simulink model "simulation_LQI"  (R2021b)
settings: Solver=FixedStepAuto  StartTime=0.0  StopTime=T  RelTol=1e-3  EnableMultiTasking=on
undefined symbols (not defined in the file or in its folder): DiscIntNeverNeededParam, discrete_eq, h, Humusoft, K_qli, MF634
libraries: sldrtlib x2, eeLuenbergerObserver x1, simulink x1
settings Model: Creator=rbabuska  LastModifiedBy=wterhaar
settings SolverCC: AlgebraicLoopSolver=TrustRegion  AutoInsertRateTranBlk=on
settings DataIOCC: LimitDataPoints=on  SaveFormat=Array  SignalLoggingSaveFormat=ModelDataLogs  SaveOutput=off  SaveTime=off  ReturnWorkspaceOutputs=off
settings OptimizationCC: DefaultParameterBehavior=Inlined  InlineInvariantSignals=on  EnhancedBackFolding=on  PassReuseOutputArgsAs=Individual arguments  ExpressionDepthLimit=2147483647  StateBitsets=on  DataBitsets=on  ZeroExternalMemoryAtStartup=off  ZeroInternalMemoryAtStartup=off  NoFixptDivByZeroProtection=on  LifeSpan=1  OptimizeBlockOrder=speed  DifferentSizesBufferReuse=on  EfficientTunableParamExpr=on
settings DebuggingCC: UnderspecifiedInitializationDetection=Classic  MergeDetectMultiDrivingBlocksExec=none  ParameterTunabilityLossMsg=error  FcnCallInpInsideContextMsg=warning  StateNameClashWarn=warning  SFUnexpectedBacktrackingDiag=warning  SFNoUnconditionalDefaultTransitionDiag=warning  SFExecutionAtInitializationDiag=none  SFMachineParentedDataDiag=warning  ArithmeticOperatorsInVariantConditions=warning
settings HardwareCC: ProdBitPerPointer=32  ProdBitPerSizeT=32  ProdBitPerPtrDiffT=32  ProdLargestAtomicFloat=None  ProdIntDivRoundTo=Floor  ProdWordSize=32  ProdHWDeviceType=Generic->Custom
settings ModelReferenceCC: PropagateSignalLabelsOutOfModel=off
settings SFSimCC: SimUseLocalCustomCode=off  MATLABDynamicMemAlloc=off  CustomCodeUndefinedFunction=UseInterfaceOnly
settings RTWCC: Description=Embedded Coder  SystemTargetFile=ert.tlc  TLCOptions=-p0  GenCodeOnly=on  TemplateMakefile=ert_default_tmf  GenerateReport=on  RTWVerbose=off  RTWUseLocalCustomCode=off  IncludeHyperlinkInReport=on  LaunchReport=on
settings CodeAppCC: ForceParamTrailComments=on  IgnoreCustomStorageClasses=off  OperatorAnnotations=on  SimulinkDataObjDesc=on  SFDataObjDesc=on  CustomSymbolStrGlobalVar=rt$N$M  CustomSymbolStrType=$N$M  CustomSymbolStrFcn=$N$M$F  CustomSymbolStrMacro=$N$M  InsertBlockDesc=on
settings ERTTargetCC: CodeReplacementLibrary=ISO_C  GenerateSampleERTMain=on  IncludeMdlTerminateFcn=off  SuppressErrorStatus=on  SupportAbsoluteTime=off  PurelyIntegerCode=on  SupportNonFinite=off  SupportComplex=off  InlinedParameterPlacement=NonHierarchical  RootIOFormat=Structure reference  ERTCustomFileTemplate=example_file_process.tlc
settings ConfigComp: CovMetricSettings=dw  CovSaveCumulativeToWorkspaceVar=on  CovSaveSingleToWorkspaceVar=on  CovExternalEMLEnable=off  CovSFcnEnable=off

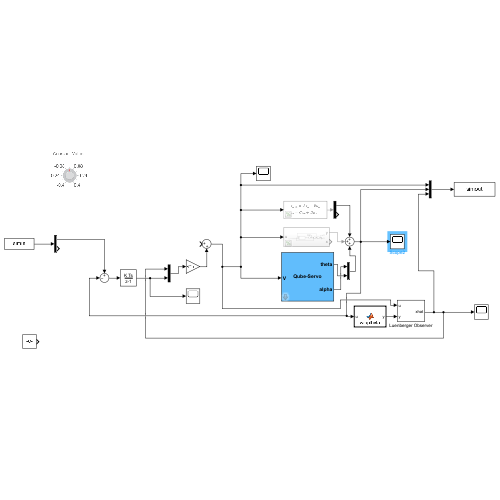
[thumbnail: Simulink's stored preview of the top-level diagram]
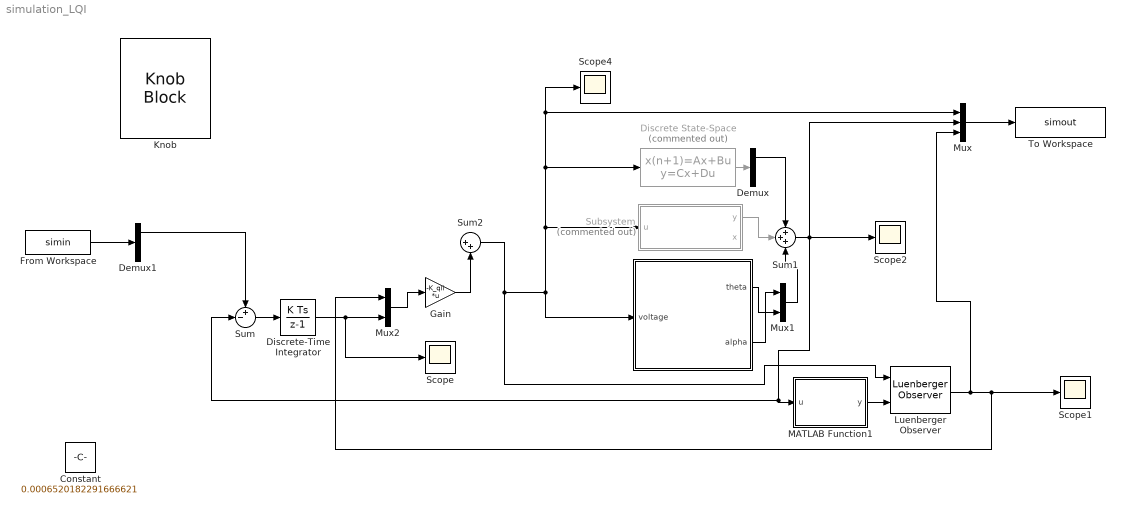
== system simulation_LQI ==
  " " : Subsystem  LoadFcn=hwinit  InitFcn=hwinit  mask{h=h}
      mask prompts: h "Sampling period [s]"
      mask Display:
      | disp('Qube-Servo')
      | port_label('output',1,'theta')
      | port_label('output',2,'alpha')
      | port_label('input',1,'V')
  Constant : Constant  Value=0.0006520182291666621
  Demux : Demux  Outputs=[2;4]
  Demux1 : Demux  Outputs=[2 2]
  Discrete State-Space : DiscreteStateSpace  Commented=on  A=discrete_eq.A  B=discrete_eq.B  C=[discrete_eq.C;eye(4)]  D=[discrete_eq.D;zeros(4,1)]  InitialCondition=[0;0;0;0]  SampleTime=h
  Discrete-Time Integrator : DiscreteIntegrator  gainval=[1;0.001]  InitialCondition=[0;0]  SampleTime=h  ICPrevOutput=DiscIntNeverNeededParam  ICPrevScaledInput=DiscIntNeverNeededParam
  From Workspace : FromWorkspace  VariableName=simin  SampleTime=h  OutputAfterFinalValue=Holding final value
  Gain : Gain  Gain=-K_qli  Multiplication=Matrix(K*u)
  Knob : KnobBlock  ScaleMin=-0.4  ScaleMax=0.4
  Luenberger Observer : eeLuenbergerObserver/Luenberger Observer  StateSpaceType=Discrete-time  Ad=discrete_eq.A  Bd=discrete_eq.B  Cd=discrete_eq.C  Dd=discrete_eq.D  A=1  B=1  C=1  D=1  ObserverDesign=Observer gain  Ld=disc  DesiredEigenvalues=pDisc  x0=[0;0;0;0]  Tsd=0.1  Ts=h
      settings: SourceProductBaseCode=PS
  MATLAB Function1 : MATLAB Function  TreatAsAtomicUnit=on
  Mux : Mux  Inputs=3
  Mux1 : Mux  Inputs=2
  Mux2 : Mux  Inputs=2
  Scope{,1..2,4} (4 alike) : Scope
  Subsystem : Subsystem  Commented=on
  Sum : Sum  Inputs=+-|
  Sum1 : Sum  Inputs=+++
  Sum2 : Sum  Inputs=|++
  To Workspace : ToWorkspace  VariableName=simout  SaveFormat=Timeseries  SampleTime=-1
  wires:
  Mux/1 -> To Workspace/1
  Luenberger Observer/1 -> Mux/3, Mux2/1, Scope1/1
  " "/2(alpha) -> Mux1/1
  " "/1(theta) -> Mux1/2
  Mux1/1 -> Sum1/3
  Subsystem/1(y) -> Sum1/2
  Demux/1 -> Sum1/1
  Sum1/1 -> Sum/2, MATLAB Function1/1(u), Mux/2, Scope2/1
  MATLAB Function1/1(y) -> Luenberger Observer/2
  Discrete State-Space/1 -> Demux/1
  Discrete-Time Integrator/1 -> Scope/1, Mux2/2
  Mux2/1 -> Gain/1
  Sum2/1 -> Luenberger Observer/1, Subsystem/1(u), Discrete State-Space/1, Mux/1, Scope4/1, " "/1(voltage)
  Sum/1 -> Discrete-Time Integrator/1
  Gain/1 -> Sum2/2
  From Workspace/1 -> Demux1/1
  Demux1/1 -> Sum/1

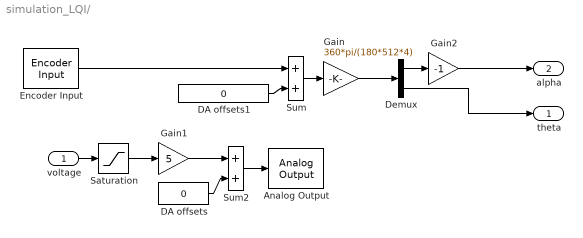
== system simulation_LQI/  ==
  voltage : Inport
  Analog Output : sldrtlib/Analog Output  SampleTime=h  MaxMissedTicks=100  ShowMissedTicks=off  YieldWhenWaiting=off  DrvName=Humusoft/MF634  DrvAddress=4294967295  DrvOptions=0  Channels=[1]  RangeMode=2  VoltRange=1  InitialValue=0  FinalValue=0
      settings: AttributesFormatString=Humusoft\nMF634 [auto]
  DA offsets : Constant  Value=0
  DA offsets1 : Constant  Value=0  SampleTime=h
  Demux : Demux  Outputs=2
  Encoder Input : sldrtlib/Encoder Input  SampleTime=h  MaxMissedTicks=100  ShowMissedTicks=off  YieldWhenWaiting=off  DrvName=Humusoft/MF634  DrvAddress=4294967295  DrvOptions=0  Channels=[1,2]  QuadMode=3  IndexPulse=1  InputFilter=Inf  DataType=1
      settings: AttributesFormatString=Humusoft\nMF634 [auto]
  Gain : Gain  Gain=360*pi/(180*512*4)  SaturateOnIntegerOverflow=on  OutDataTypeStr=Inherit: Same as input  ParamDataTypeStr=Inherit: Same as input
  Gain1 : Gain  Gain=5  SaturateOnIntegerOverflow=on  OutDataTypeStr=Inherit: Same as input  ParamDataTypeStr=Inherit: Same as input
  Gain2 : Gain  Gain=-1  SaturateOnIntegerOverflow=on  OutDataTypeStr=Inherit: Same as input  ParamDataTypeStr=Inherit: Same as input
  Saturation : Saturate  UpperLimit=1  LowerLimit=-1
  Sum : Sum  InputSameDT=on  SaturateOnIntegerOverflow=on  OutDataTypeStr=Inherit: Same as first input
  Sum2 : Sum  InputSameDT=on  SaturateOnIntegerOverflow=on  OutDataTypeStr=Inherit: Same as first input
  theta : Outport  Tag=Cable length
  alpha : Outport  Tag=Cable length  Port=2
  wires:
  Sum/1 -> Gain/1
  DA offsets1/1 -> Sum/2
  Gain1/1 -> Sum2/1
  Sum2/1 -> Analog Output/1
  DA offsets/1 -> Sum2/2
  voltage/1 -> Saturation/1
  Encoder Input/1 -> Sum/1
  Saturation/1 -> Gain1/1
  Demux/1 -> Gain2/1
  Gain/1 -> Demux/1
  Gain2/1 -> alpha/1
  Demux/2 -> theta/1

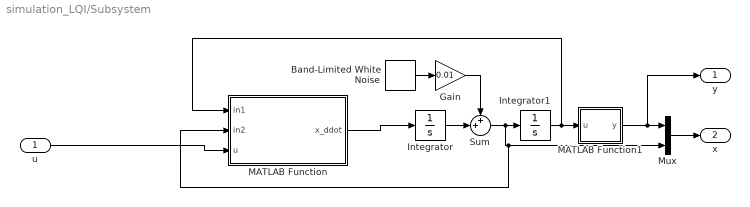
== system simulation_LQI/Subsystem ==
  u : Inport
  Band-Limited White Noise : simulink/Sources/Band-Limited White Noise  Cov=1  Ts=h  seed=[23341]
  Gain : Gain  Gain=0.01
  Integrator : Integrator
  Integrator1 : Integrator  InitialCondition=[0;pi]
  MATLAB Function : MATLAB Function  TreatAsAtomicUnit=on
  MATLAB Function1 : MATLAB Function  TreatAsAtomicUnit=on
  Mux : Mux  Inputs=2
  Sum : Sum  Inputs=++|
  y : Outport  PortDimensions=2
  x : Outport  Port=2  PortDimensions=4
  wires:
  Integrator/1 -> Sum/2
  Sum/1 -> MATLAB Function/2(in2), Mux/2, Integrator1/1
  MATLAB Function1/1(y) -> y/1, Mux/1
  MATLAB Function/1(x_ddot) -> Integrator/1
  u/1 -> MATLAB Function/3(u)
  Mux/1 -> x/1
  Band-Limited White Noise/1 -> Gain/1
  Gain/1 -> Sum/1
  Integrator1/1 -> MATLAB Function/1(in1), MATLAB Function1/1(u)

== matlab function simulation_LQI/Subsystem/MATLAB Function ==
  data: in1 input; in2 input; x_ddot output; u input
function x_ddot = generated_nonlinfit(in1,in2,u)
%GENERATED_NONLINFIT
%    X_DDOT = GENERATED_NONLINFIT(IN1,IN2,U)

%    This function was generated by the Symbolic Math Toolbox version 9.0.
%    26-Oct-2022 21:30:39

alpha = in1(1,:);
alpha_dot = in2(1,:);
theta = in1(2,:);
theta_dot = in2(2,:);
t2 = cos(theta);
t3 = sin(theta);
t4 = theta_dot.^2;
t5 = t2.^2;
t6 = t5.*5.202e-4;
t7 = t6-1.025001736928224e-3;
t8 = 1.0./t7;
et1 = alpha.*(-1.861031175243817e-2)-alpha_dot.*2.355807420816275e-3+u.*7.776000919769337e-1;
et2 = t2.*t3.*6.32066282169313e-2+t3.*t4.*5.283326721496806e-4+t2.*theta_dot.*5.2382775346984e-5;
et3 = t3.*1.270331445249629e-4;
et4 = theta_dot.*1.052792857172148e-7-alpha.*t2.*1.898251798748694e-5;
et5 = alpha_dot.*t2.*(-2.402923569232601e-6)+t2.*u.*7.931520938164723e-4+t2.*t3.*t4.*5.388993255926742e-7;
x_ddot = [t8.*(et1+et2).*(-9.498560782889175e-1);t8.*(et3+et4+et5).*9.653008925700381e+2];

== matlab function simulation_LQI/MATLAB Function1 ==
  data: u input; y output
function y = wraptheta(u)

y=u;
y(2)=wrapToPi(u(2));

== matlab function simulation_LQI/Subsystem/MATLAB Function1 ==
  data: u input; y output
function y = wrap(u)
y=[
    u(1)
    wrapToPi(u(2)-pi)
];
